simulink model "STP_1b"  (R2023a)
settings: Solver=ode4  StartTime=0.0  StopTime=30  FixedStep=0.005  RelTol=1e-3
InitFcn:
  | STP
values from neighbouring files (symbols this model uses):
  K_scheduled = zeros(length(V_op), 2)    [CAL3.m]    (also in CUB.m; DLC2.m; MUS.m; OHZ.m)
  V_op = 5:5:85    [CAL3.m]    (also in CUB.m; DLC2.m; MUS.m; OHZ.m)
  X_track = [linspace(0, runway_length, 200)'; runway_length + R_track * cos(theta_circ(2:end))]    [CAL3.m]    (also in CUB.m = [0; 5000]; DLC2.m = 0:0.1:total_track_length; MUS.m = [0; 2000]; OHZ.m = [0; 2000])
  Y_track = [zeros(200, 1); R_track + R_track * sin(theta_circ(2:end))]    [CAL3.m]    (also in CUB.m = [0; 0]; DLC2.m = zeros(size(X_track)); MUS.m = [0; 0]; OHZ.m = [0; 0])
libraries: simulink x2, slpidlib x2
(part 1 of 3)
settings Model: NumberOfSteps=1000  SnapshotBufferSize=1000  SnapshotInterval=1000  Creator=KBISWAS  LastModifiedBy=KBISWAS

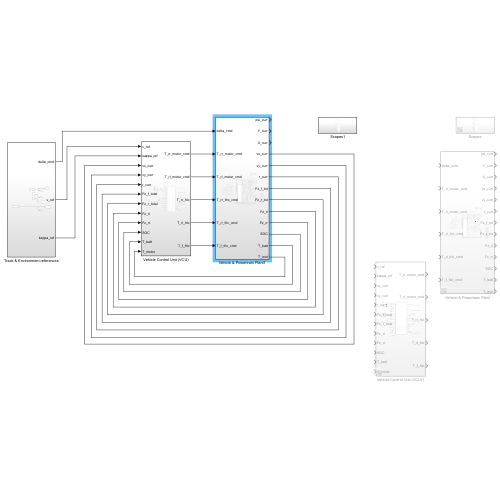
[thumbnail: Simulink's stored preview of the top-level diagram]
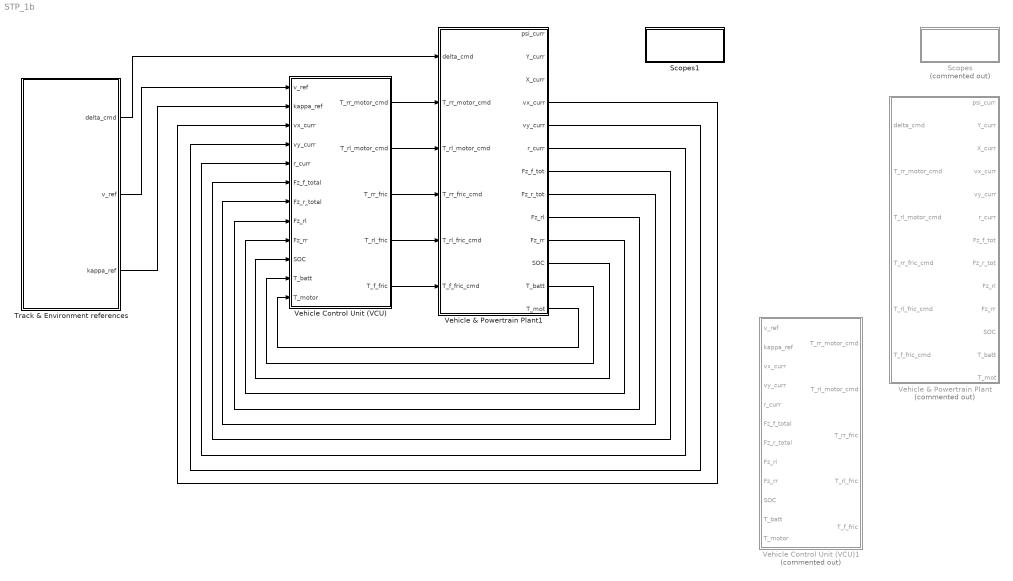
== system STP_1b ==
  Scopes : Subsystem  Commented=on
  Scopes1 : Subsystem
  Track & Environment references : Subsystem
  Vehicle & Powertrain Plant : Subsystem  Commented=on
  Vehicle & Powertrain Plant1 : Subsystem
  Vehicle Control Unit (VCU) : Subsystem
  Vehicle Control Unit (VCU)1 : Subsystem  Commented=on
  wires:
  Track & Environment references/2(v_ref) -> Vehicle Control Unit (VCU)/1(v_ref)
  Vehicle Control Unit (VCU)/1(T_rr_motor_cmd) -> Vehicle & Powertrain Plant1/2(T_rr_motor_cmd)
  Track & Environment references/3(kappa_ref) -> Vehicle Control Unit (VCU)/2(kappa_ref)
  Track & Environment references/1(delta_cmd) -> Vehicle & Powertrain Plant1/1(delta_cmd)
  Vehicle Control Unit (VCU)/2(T_rl_motor_cmd) -> Vehicle & Powertrain Plant1/3(T_rl_motor_cmd)
  Vehicle Control Unit (VCU)/3(T_rr_fric) -> Vehicle & Powertrain Plant1/4(T_rr_fric_cmd)
  Vehicle Control Unit (VCU)/4(T_rl_fric) -> Vehicle & Powertrain Plant1/5(T_rl_fric_cmd)
  Vehicle Control Unit (VCU)/5(T_f_fric) -> Vehicle & Powertrain Plant1/6(T_f_fric_cmd)
  Vehicle & Powertrain Plant1/4(vx_curr) -> Vehicle Control Unit (VCU)/3(vx_curr)
  Vehicle & Powertrain Plant1/5(vy_curr) -> Vehicle Control Unit (VCU)/4(vy_curr)
  Vehicle & Powertrain Plant1/6(r_curr) -> Vehicle Control Unit (VCU)/5(r_curr)
  Vehicle & Powertrain Plant1/7(Fz_f_tot) -> Vehicle Control Unit (VCU)/6(Fz_f_total)
  Vehicle & Powertrain Plant1/8(Fz_r_tot) -> Vehicle Control Unit (VCU)/7(Fz_r_total)
  Vehicle & Powertrain Plant1/9(Fz_rl) -> Vehicle Control Unit (VCU)/8(Fz_rl)
  Vehicle & Powertrain Plant1/10(Fz_rr) -> Vehicle Control Unit (VCU)/9(Fz_rr)
  Vehicle & Powertrain Plant1/11(SOC) -> Vehicle Control Unit (VCU)/10(SOC)
  Vehicle & Powertrain Plant1/12(T_batt) -> Vehicle Control Unit (VCU)/11(T_batt)
  Vehicle & Powertrain Plant1/13(T_mot) -> Vehicle Control Unit (VCU)/12(T_motor)

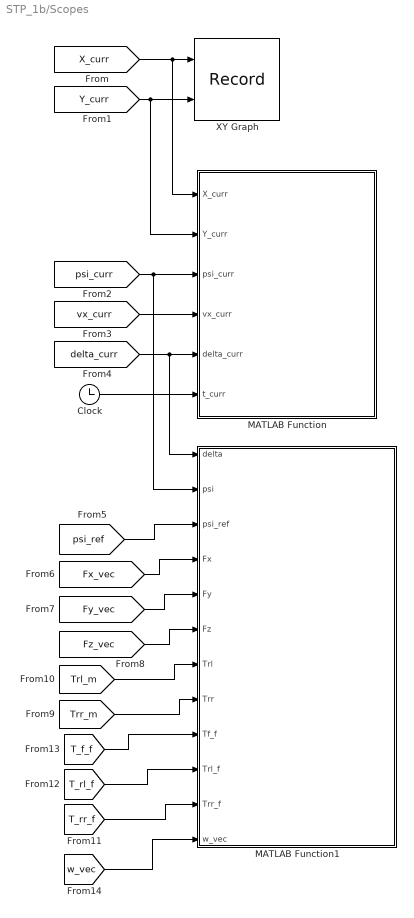
== system STP_1b/Scopes ==
  Clock : Clock
  MATLAB Function : MATLAB Function  TreatAsAtomicUnit=on
  MATLAB Function1 : MATLAB Function  TreatAsAtomicUnit=on
  XY Graph : Record  FileSettingsInternal="{\"entries\":[{\"content\":{\"excelSettings\":{\"content\":{},\"type\":\"Streamout.ExcelSettings\"}},\"type\":\"Streamout.FileSettingStorage\",\"uuid\":\"\"}],\"packageUris\":[\"http:\\/\\/schema.mathworks.com\\/mf0\\/streamout_blocks\\/R2020a\"],\"version\":\"1.0\"}"  Layout=[1 1]  SignalsInternal="{\"entries\":[{\"content\":{},\"type\":\"RecordBlkView.InputSignals\",\"uuid\":\"\"}],\"packageUris\":[\"http:\\/\\/schema.mathworks.com\\/mf0\\/streamout_blocks\\/R2020a\"],\"version\":\"1.0\"}"  VisualizationBindings="{\"xyplotplugin\":{\"info\":[{\"series\":[],\"subplotID\":1}]}}"  CompatibilityTag=XY
  wires:
  [X_curr] -> MATLAB Function/1(X_curr), XY Graph/1
  [Y_curr] -> MATLAB Function/2(Y_curr), XY Graph/2
  [psi_curr] -> MATLAB Function/3(psi_curr), MATLAB Function1/2(psi)
  [vx_curr] -> MATLAB Function/4(vx_curr)
  [delta_curr] -> MATLAB Function1/1(delta), MATLAB Function/5(delta_curr)
  Clock/1 -> MATLAB Function/6(t_curr)
  [psi_ref] -> MATLAB Function1/3(psi_ref)
  [Fx_vec] -> MATLAB Function1/4(Fx)
  [Fy_vec] -> MATLAB Function1/5(Fy)
  [Fz_vec] -> MATLAB Function1/6(Fz)
  [Trr_m] -> MATLAB Function1/8(Trr)
  [Trl_m] -> MATLAB Function1/7(Trl)
  [T_f_f] -> MATLAB Function1/9(Tf_f)
  [T_rr_f] -> MATLAB Function1/11(Trr_f)
  [T_rl_f] -> MATLAB Function1/10(Trl_f)
  [w_vec] -> MATLAB Function1/12(w_vec)

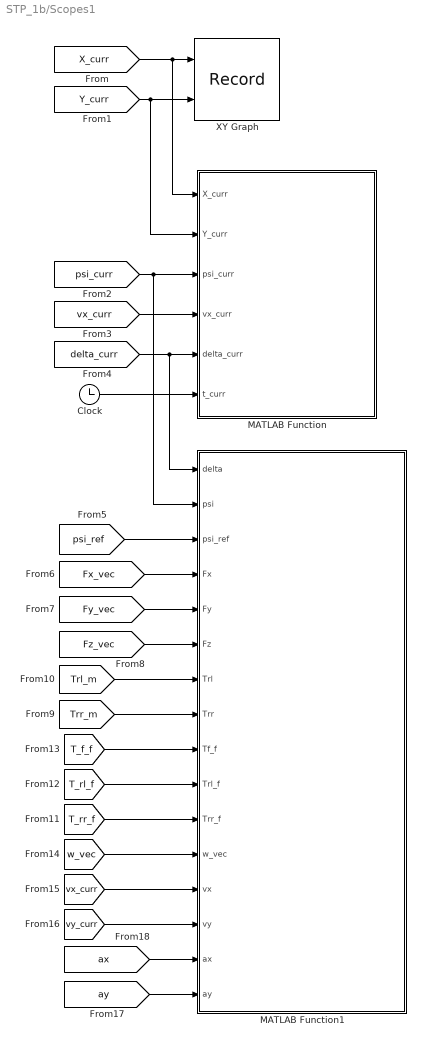
== system STP_1b/Scopes1 ==
  Clock : Clock
  MATLAB Function : MATLAB Function  TreatAsAtomicUnit=on
  MATLAB Function1 : MATLAB Function  TreatAsAtomicUnit=on
  XY Graph : Record  FileSettingsInternal="{\"entries\":[{\"content\":{\"excelSettings\":{\"content\":{},\"type\":\"Streamout.ExcelSettings\"}},\"type\":\"Streamout.FileSettingStorage\",\"uuid\":\"\"}],\"packageUris\":[\"http:\\/\\/schema.mathworks.com\\/mf0\\/streamout_blocks\\/R2020a\"],\"version\":\"1.0\"}"  Layout=[1 1]  SignalsInternal="{\"entries\":[{\"content\":{\"signals\":[{\"content\":{\"blockPath\":[],\"dimensions\":[1],\"domain\":\"\",\"lineColor\":\"#fe330a\",\"port\":1,\"sid\":[\"\"],\"signalID\":421428,\"signalName\":\"From\"},\"type\":\"RecordBlkView.Signal\",\"uuid\":\"\"},{\"content\":{\"blockPath\":[],\"dimensions\":[1],\"domain\":\"\",\"lineColor\":\"#22b573\",\"port\":2,\"sid\":[\"\"],\"signalID\":421432,\"signalName\":\"From1\"},\"type\":\"RecordBlkView.Signal\",\"uuid\":\"\"}]},\"type\":\"RecordBlkView.InputSignals\",\"uuid\":\"\"}],\"packageUris\":[\"http:\\/\\/schema.mathworks.com\\/mf0\\/streamout_blocks\\/R2020a\"],\"version\":\"1.0\"}"  VisualizationBindings="{\"xyplotplugin\":{\"info\":[{\"series\":[],\"subplotID\":1}]}}"  CompatibilityTag=XY
  wires:
  [X_curr] -> MATLAB Function/1(X_curr), XY Graph/1
  [Y_curr] -> MATLAB Function/2(Y_curr), XY Graph/2
  [psi_curr] -> MATLAB Function1/2(psi), MATLAB Function/3(psi_curr)
  [vx_curr] -> MATLAB Function/4(vx_curr)
  [delta_curr] -> MATLAB Function1/1(delta), MATLAB Function/5(delta_curr)
  Clock/1 -> MATLAB Function/6(t_curr)
  [psi_ref] -> MATLAB Function1/3(psi_ref)
  [Fx_vec] -> MATLAB Function1/4(Fx)
  [Fy_vec] -> MATLAB Function1/5(Fy)
  [Fz_vec] -> MATLAB Function1/6(Fz)
  [Trr_m] -> MATLAB Function1/8(Trr)
  [Trl_m] -> MATLAB Function1/7(Trl)
  [T_f_f] -> MATLAB Function1/9(Tf_f)
  [T_rr_f] -> MATLAB Function1/11(Trr_f)
  [T_rl_f] -> MATLAB Function1/10(Trl_f)
  [w_vec] -> MATLAB Function1/12(w_vec)
  [vx_curr] -> MATLAB Function1/13(vx)
  [vy_curr] -> MATLAB Function1/14(vy)
  [ax] -> MATLAB Function1/15(ax)
  [ay] -> MATLAB Function1/16(ay)

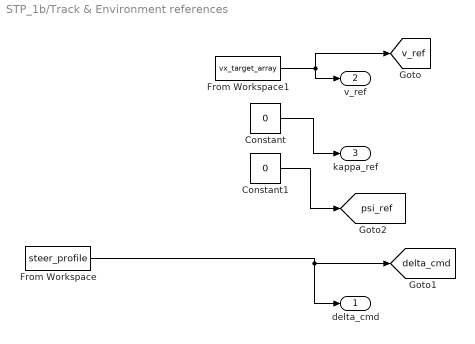
== system STP_1b/Track & Environment references ==
  Constant : Constant  Value=0
  Constant1 : Constant  Value=0
  From Workspace : FromWorkspace  VariableName=steer_profile
  From Workspace1 : FromWorkspace  VariableName=vx_target_array
  delta_cmd : Outport
  v_ref : Outport  Port=2
  kappa_ref : Outport  Port=3
  tag scope: delta_cmd=global, psi_ref=global, v_ref=global
  wires:
  From Workspace/1 -> delta_cmd/1, [delta_cmd]
  From Workspace1/1 -> v_ref/1, [v_ref]
  Constant1/1 -> [psi_ref]
  Constant/1 -> kappa_ref/1

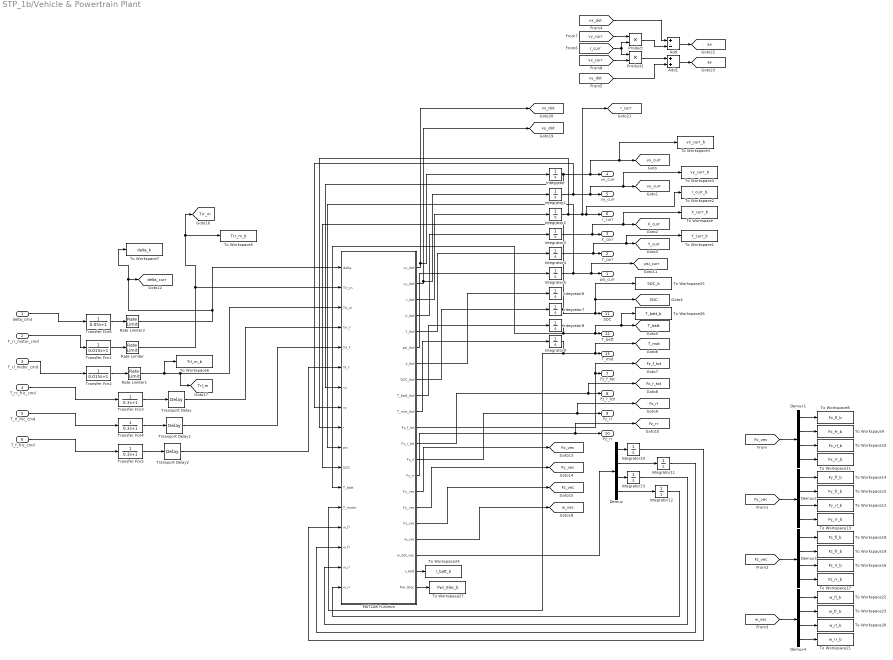
== system STP_1b/Vehicle & Powertrain Plant ==
  delta_cmd : Inport
  T_rr_motor_cmd : Inport  Port=2
  T_rl_motor_cmd : Inport  Port=3
  T_rr_fric_cmd : Inport  Port=4
  T_rl_fric_cmd : Inport  Port=5
  T_f_fric_cmd : Inport  Port=6
  Add : Sum  Inputs=+-
  Add1 : Sum
  Demux{,1..4} (5 alike) : Demux
  Integrator : Integrator  InitialCondition=5
  Integrator{1..6,10..13} (10 alike) : Integrator
  Integrator7 : Integrator  InitialCondition=0.9
  Integrator8 : Integrator  InitialCondition=30
  Integrator9 : Integrator  InitialCondition=30
  MATLAB Function : MATLAB Function  TreatAsAtomicUnit=on
  Product : Product
  Product1 : Product
  Rate Limiter : RateLimiter  RisingSlewLimit=500  FallingSlewLimit=-500  SampleTimeMode=inherited
  Rate Limiter1 : RateLimiter  RisingSlewLimit=500  FallingSlewLimit=-500  SampleTimeMode=inherited
  Rate Limiter2 : RateLimiter  RisingSlewLimit=0.05  FallingSlewLimit=-0.05  SampleTimeMode=inherited
  To Workspace : ToWorkspace  VariableName=X_curr_b  SaveFormat=Timeseries  SampleTime=-1
  To Workspace1 : ToWorkspace  VariableName=Y_curr_b  SaveFormat=Timeseries  SampleTime=-1
  To Workspace10 : ToWorkspace  VariableName=Fx_rl_b  SaveFormat=Timeseries  SampleTime=-1
  To Workspace11 : ToWorkspace  VariableName=Fx_rr_b  SaveFormat=Timeseries  SampleTime=-1
  To Workspace12 : ToWorkspace  VariableName=Fy_rl_b  SaveFormat=Timeseries  SampleTime=-1
  To Workspace13 : ToWorkspace  VariableName=Fy_rr_b  SaveFormat=Timeseries  SampleTime=-1
  To Workspace14 : ToWorkspace  VariableName=Fy_fl_b  SaveFormat=Timeseries  SampleTime=-1
  To Workspace15 : ToWorkspace  VariableName=Fy_fr_b  SaveFormat=Timeseries  SampleTime=-1
  To Workspace16 : ToWorkspace  VariableName=Fz_rl_b  SaveFormat=Timeseries  SampleTime=-1
  To Workspace17 : ToWorkspace  VariableName=Fz_rr_b  SaveFormat=Timeseries  SampleTime=-1
  To Workspace18 : ToWorkspace  VariableName=Fz_fl_b  SaveFormat=Timeseries  SampleTime=-1
  To Workspace19 : ToWorkspace  VariableName=Fz_fr_b  SaveFormat=Timeseries  SampleTime=-1
  To Workspace2 : ToWorkspace  VariableName=r_curr_b  SaveFormat=Timeseries  SampleTime=-1
  To Workspace20 : ToWorkspace  VariableName=w_rl_b  SaveFormat=Timeseries  SampleTime=-1
  To Workspace21 : ToWorkspace  VariableName=w_rr_b  SaveFormat=Timeseries  SampleTime=-1
  To Workspace22 : ToWorkspace  VariableName=w_fl_b  SaveFormat=Timeseries  SampleTime=-1
  To Workspace23 : ToWorkspace  VariableName=w_fr_b  SaveFormat=Timeseries  SampleTime=-1
  To Workspace24 : ToWorkspace  VariableName=I_batt_b  SaveFormat=Timeseries  SampleTime=-1
  To Workspace25 : ToWorkspace  VariableName=SOC_b  SaveFormat=Timeseries  SampleTime=-1
  To Workspace26 : ToWorkspace  VariableName=T_batt_b  SaveFormat=Timeseries  SampleTime=-1
  To Workspace27 : ToWorkspace  VariableName=Pwr_Elec_b  SaveFormat=Timeseries  SampleTime=-1
  To Workspace3 : ToWorkspace  VariableName=vx_curr_b  SaveFormat=Timeseries  SampleTime=-1
  To Workspace4 : ToWorkspace  VariableName=vy_curr_b  SaveFormat=Timeseries  SampleTime=-1
  To Workspace5 : ToWorkspace  VariableName=Trr_m_b  SaveFormat=Timeseries  SampleTime=-1
  To Workspace6 : ToWorkspace  VariableName=Trl_m_b  SaveFormat=Timeseries  SampleTime=-1
  To Workspace7 : ToWorkspace  VariableName=delta_b  SaveFormat=Timeseries  SampleTime=-1
  To Workspace8 : ToWorkspace  VariableName=Fx_fl_b  SaveFormat=Timeseries  SampleTime=-1
  To Workspace9 : ToWorkspace  VariableName=Fx_fr_b  SaveFormat=Timeseries  SampleTime=-1
  Transfer Fcn1 : TransferFcn  Denominator=[0.015 1]
  Transfer Fcn2 : TransferFcn  Denominator=[0.015 1]
  Transfer Fcn3 : TransferFcn  Denominator=[0.3 1]
  Transfer Fcn4 : TransferFcn  Denominator=[0.3 1]
  Transfer Fcn5 : TransferFcn  Denominator=[0.3 1]
  Transfer Fcn6 : TransferFcn  Numerator=1  Denominator=[0.05 1]
  Transport Delay : TransportDelay  DelayTime=0.03
  Transport Delay1 : TransportDelay  DelayTime=0.03
  Transport Delay2 : TransportDelay  DelayTime=0.03
  psi_curr : Outport
  Y_curr : Outport  Port=2
  X_curr : Outport  Port=3
  vx_curr : Outport  Port=4
  vy_curr : Outport  Port=5
  r_curr : Outport  Port=6
  Fz_f_tot : Outport  Port=7
  Fz_r_tot : Outport  Port=8
  Fz_rl : Outport  Port=9
  Fz_rr : Outport  Port=10
  SOC : Outport  Port=11
  T_batt : Outport  Port=12
  T_mot : Outport  Port=13
  tag scope: Fx_vec=global, Fy_vec=global, Fz_f_tot=global, Fz_r_tot=global, Fz_rl=global, Fz_rr=global, Fz_vec=global, SOC=global, T_batt=global, T_mot=global, Trl_m=global, Trr_m=global, X_curr=global, Y_curr=global, ax=global, ay=global, delta_curr=global, psi_curr=global, r_curr=global, vx_curr=global, vx_dot=global, vy_curr=global, vy_dot=global, w_vec=global
  wires:
  T_rr_fric_cmd/1 -> Transfer Fcn3/1
  T_rl_fric_cmd/1 -> Transfer Fcn4/1
  T_f_fric_cmd/1 -> Transfer Fcn5/1
  Rate Limiter2/1 -> MATLAB Function/1(delta), To Workspace7/1, [delta_curr]
  Rate Limiter/1 -> To Workspace5/1, [Trr_m], MATLAB Function/2(Trr_m)
  Rate Limiter1/1 -> To Workspace6/1, MATLAB Function/3(Trl_m), [Trl_m]
  Transfer Fcn3/1 -> Transport Delay/1
  Transfer Fcn4/1 -> Transport Delay1/1
  Transfer Fcn5/1 -> Transport Delay2/1
  MATLAB Function/3(r_dot) -> Integrator2/1
  MATLAB Function/4(X_dot) -> Integrator3/1
  MATLAB Function/5(Y_dot) -> Integrator4/1
  MATLAB Function/6(psi_dot) -> Integrator5/1
  MATLAB Function/7(s_dot) -> Integrator6/1
  MATLAB Function/8(SOC_dot) -> Integrator7/1
  Integrator/1 -> MATLAB Function/7(vx), To Workspace3/1, [vx_curr], vx_curr/1
  Integrator1/1 -> MATLAB Function/8(vy), To Workspace4/1, [vy_curr], vy_curr/1
  Integrator5/1 -> MATLAB Function/10(psi), [psi_curr], psi_curr/1
  Integrator8/1 -> MATLAB Function/12(T_batt), To Workspace26/1, [T_batt], T_batt/1
  Integrator9/1 -> MATLAB Function/13(T_motor), [T_mot], T_mot/1
  Integrator4/1 -> To Workspace1/1, [Y_curr], Y_curr/1
  Integrator3/1 -> To Workspace/1, [X_curr], X_curr/1
  MATLAB Function/11(Fz_f_tot) -> [Fz_f_tot], Fz_f_tot/1
  Integrator7/1 -> MATLAB Function/11(SOC), To Workspace25/1, [SOC], SOC/1
  MATLAB Function/14(Fz_rr) -> [Fz_rr], Fz_rr/1
  MATLAB Function/15(Fx_vec) -> [Fx_vec]
  MATLAB Function/17(Fz_vec) -> [Fz_vec]
  MATLAB Function/9(T_batt_dot) -> Integrator8/1
  MATLAB Function/10(T_mot_dot) -> Integrator9/1
  MATLAB Function/12(Fz_r_tot) -> [Fz_r_tot], Fz_r_tot/1
  MATLAB Function/13(Fz_rl) -> [Fz_rl], Fz_rl/1
  MATLAB Function/16(Fy_vec) -> [Fy_vec]
  MATLAB Function/18(w_vec) -> [w_vec]
  Demux/4 -> Integrator12/1
  Demux/3 -> Integrator13/1
  Demux/2 -> Integrator11/1
  Demux/1 -> Integrator10/1
  MATLAB Function/19(w_dot_vec) -> Demux/1
  Integrator10/1 -> MATLAB Function/14(w_fl)
  Integrator11/1 -> MATLAB Function/15(w_fr)
  Integrator12/1 -> MATLAB Function/17(w_rr)
  Integrator13/1 -> MATLAB Function/16(w_rl)
  Demux1/2 -> To Workspace9/1
  [w_vec] -> Demux4/1
  Demux3/2 -> To Workspace19/1
  Demux3/4 -> To Workspace17/1
  Demux3/3 -> To Workspace16/1
  [Fy_vec] -> Demux2/1
  Demux2/1 -> To Workspace14/1
  Demux2/3 -> To Workspace12/1
  [Fz_vec] -> Demux3/1
  Demux2/4 -> To Workspace13/1
  Demux2/2 -> To Workspace15/1
  Demux1/4 -> To Workspace11/1
  Demux1/1 -> To Workspace8/1
  Demux1/3 -> To Workspace10/1
  [Fx_vec] -> Demux1/1
  Demux3/1 -> To Workspace18/1
  Demux4/1 -> To Workspace22/1
  Demux4/4 -> To Workspace21/1
  Demux4/3 -> To Workspace20/1
  Demux4/2 -> To Workspace23/1
  Transfer Fcn1/1 -> Rate Limiter/1
  Transfer Fcn2/1 -> Rate Limiter1/1
  Product1/1 -> Add1/1
  [vy_curr] -> Product/1
  Product/1 -> Add/2
  [vx_curr] -> Product1/2
  Integrator2/1 -> [r_curr], To Workspace2/1, r_curr/1, MATLAB Function/9(r)
  MATLAB Function/1(vx_dot) -> [vx_dot], Integrator/1
  [r_curr] -> Product1/1, Product/2
  [vy_dot] -> Add1/2
  Add/1 -> [ax]
  Add1/1 -> [ay]
  [vx_dot] -> Add/1
  MATLAB Function/2(vy_dot) -> [vy_dot], Integrator1/1
  T_rr_motor_cmd/1 -> Transfer Fcn1/1
  T_rl_motor_cmd/1 -> Transfer Fcn2/1
  MATLAB Function/20(I_batt) -> To Workspace24/1
  MATLAB Function/21(Pwr_Elec) -> To Workspace27/1
  Transfer Fcn6/1 -> Rate Limiter2/1
  delta_cmd/1 -> Transfer Fcn6/1
  Transport Delay1/1 -> MATLAB Function/5(Trl_f)
  Transport Delay2/1 -> MATLAB Function/6(Tf_f)
  Transport Delay/1 -> MATLAB Function/4(Trr_f)

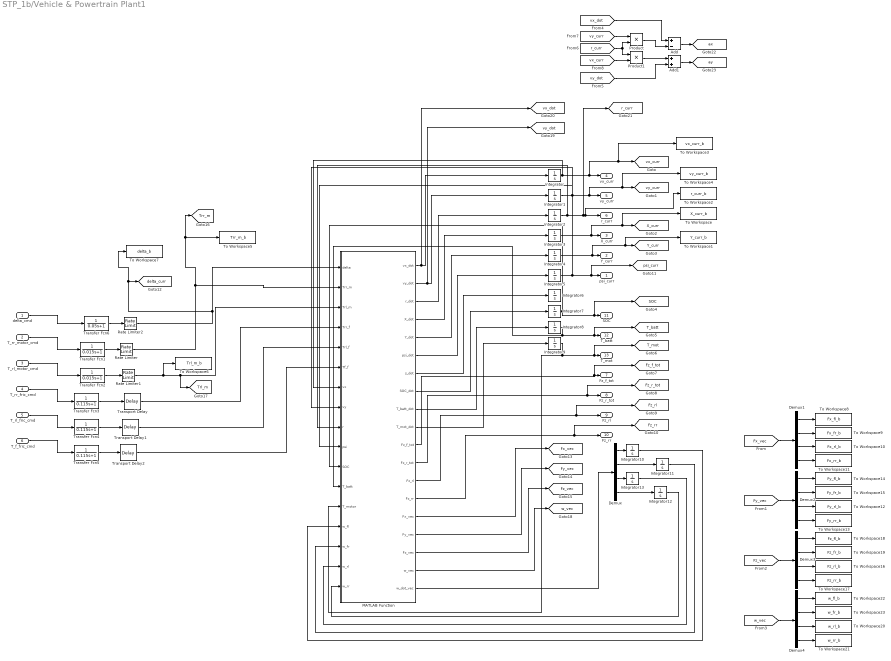
== system STP_1b/Vehicle & Powertrain Plant1 ==
  delta_cmd : Inport
  T_rr_motor_cmd : Inport  Port=2
  T_rl_motor_cmd : Inport  Port=3
  T_rr_fric_cmd : Inport  Port=4
  T_rl_fric_cmd : Inport  Port=5
  T_f_fric_cmd : Inport  Port=6
  Add : Sum  Inputs=+-
  Add1 : Sum
  Demux{,1..4} (5 alike) : Demux
  Integrator : Integrator  InitialCondition=5
  Integrator{1..6,10..13} (10 alike) : Integrator
  Integrator7 : Integrator  InitialCondition=0.9
  Integrator8 : Integrator  InitialCondition=30
  Integrator9 : Integrator  InitialCondition=30
  MATLAB Function : MATLAB Function  TreatAsAtomicUnit=on
  Product : Product
  Product1 : Product
  Rate Limiter : RateLimiter  RisingSlewLimit=500  FallingSlewLimit=-500  SampleTimeMode=inherited
  Rate Limiter1 : RateLimiter  RisingSlewLimit=500  FallingSlewLimit=-500  SampleTimeMode=inherited
  Rate Limiter2 : RateLimiter  RisingSlewLimit=0.05  FallingSlewLimit=-0.05  SampleTimeMode=inherited
  To Workspace : ToWorkspace  VariableName=X_curr_b  SaveFormat=Timeseries  SampleTime=-1
  To Workspace1 : ToWorkspace  VariableName=Y_curr_b  SaveFormat=Timeseries  SampleTime=-1
  To Workspace10 : ToWorkspace  VariableName=Fx_rl_b  SaveFormat=Timeseries  SampleTime=-1
  To Workspace11 : ToWorkspace  VariableName=Fx_rr_b  SaveFormat=Timeseries  SampleTime=-1
  To Workspace12 : ToWorkspace  VariableName=Fy_rl_b  SaveFormat=Timeseries  SampleTime=-1
  To Workspace13 : ToWorkspace  VariableName=Fy_rr_b  SaveFormat=Timeseries  SampleTime=-1
  To Workspace14 : ToWorkspace  VariableName=Fy_fl_b  SaveFormat=Timeseries  SampleTime=-1
  To Workspace15 : ToWorkspace  VariableName=Fy_fr_b  SaveFormat=Timeseries  SampleTime=-1
  To Workspace16 : ToWorkspace  VariableName=Fz_rl_b  SaveFormat=Timeseries  SampleTime=-1
  To Workspace17 : ToWorkspace  VariableName=Fz_rr_b  SaveFormat=Timeseries  SampleTime=-1
  To Workspace18 : ToWorkspace  VariableName=Fz_fl_b  SaveFormat=Timeseries  SampleTime=-1
  To Workspace19 : ToWorkspace  VariableName=Fz_fr_b  SaveFormat=Timeseries  SampleTime=-1
  To Workspace2 : ToWorkspace  VariableName=r_curr_b  SaveFormat=Timeseries  SampleTime=-1
  To Workspace20 : ToWorkspace  VariableName=w_rl_b  SaveFormat=Timeseries  SampleTime=-1
  To Workspace21 : ToWorkspace  VariableName=w_rr_b  SaveFormat=Timeseries  SampleTime=-1
  To Workspace22 : ToWorkspace  VariableName=w_fl_b  SaveFormat=Timeseries  SampleTime=-1
  To Workspace23 : ToWorkspace  VariableName=w_fr_b  SaveFormat=Timeseries  SampleTime=-1
  To Workspace3 : ToWorkspace  VariableName=vx_curr_b  SaveFormat=Timeseries  SampleTime=-1
  To Workspace4 : ToWorkspace  VariableName=vy_curr_b  SaveFormat=Timeseries  SampleTime=-1
  To Workspace5 : ToWorkspace  VariableName=Trr_m_b  SaveFormat=Timeseries  SampleTime=-1
  To Workspace6 : ToWorkspace  VariableName=Trl_m_b  SaveFormat=Timeseries  SampleTime=-1
  To Workspace7 : ToWorkspace  VariableName=delta_b  SaveFormat=Timeseries  SampleTime=-1
  To Workspace8 : ToWorkspace  VariableName=Fx_fl_b  SaveFormat=Timeseries  SampleTime=-1
  To Workspace9 : ToWorkspace  VariableName=Fx_fr_b  SaveFormat=Timeseries  SampleTime=-1
  Transfer Fcn1 : TransferFcn  Denominator=[0.015 1]
  Transfer Fcn2 : TransferFcn  Denominator=[0.015 1]
  Transfer Fcn3 : TransferFcn  Denominator=[0.115 1]
  Transfer Fcn4 : TransferFcn  Denominator=[0.115 1]
  Transfer Fcn5 : TransferFcn  Denominator=[0.115 1]
  Transfer Fcn6 : TransferFcn  Numerator=1  Denominator=[0.05 1]
  Transport Delay : TransportDelay  DelayTime=0.05
  Transport Delay1 : TransportDelay  DelayTime=0.05
  Transport Delay2 : TransportDelay  DelayTime=0.05
  psi_curr : Outport
  Y_curr : Outport  Port=2
  X_curr : Outport  Port=3
  vx_curr : Outport  Port=4
  vy_curr : Outport  Port=5
  r_curr : Outport  Port=6
  Fz_f_tot : Outport  Port=7
  Fz_r_tot : Outport  Port=8
  Fz_rl : Outport  Port=9
  Fz_rr : Outport  Port=10
  SOC : Outport  Port=11
  T_batt : Outport  Port=12
  T_mot : Outport  Port=13
  tag scope: Fx_vec=global, Fy_vec=global, Fz_f_tot=global, Fz_r_tot=global, Fz_rl=global, Fz_rr=global, Fz_vec=global, SOC=global, T_batt=global, T_mot=global, Trl_m=global, Trr_m=global, X_curr=global, Y_curr=global, ax=global, ay=global, delta_curr=global, psi_curr=global, r_curr=global, vx_curr=global, vx_dot=global, vy_curr=global, vy_dot=global, w_vec=global
  wires:
  Demux4/2 -> To Workspace23/1
  Demux4/3 -> To Workspace20/1
  Demux4/4 -> To Workspace21/1
  Demux4/1 -> To Workspace22/1
  Demux3/1 -> To Workspace18/1
  [Fx_vec] -> Demux1/1
  Demux1/3 -> To Workspace10/1
  Demux1/1 -> To Workspace8/1
  Demux1/4 -> To Workspace11/1
  Demux2/2 -> To Workspace15/1
  Demux2/4 -> To Workspace13/1
  [Fz_vec] -> Demux3/1
  Demux2/3 -> To Workspace12/1
  Demux2/1 -> To Workspace14/1
  [Fy_vec] -> Demux2/1
  Demux3/3 -> To Workspace16/1
  Demux3/4 -> To Workspace17/1
  Demux3/2 -> To Workspace19/1
  [w_vec] -> Demux4/1
  Demux1/2 -> To Workspace9/1
  Integrator13/1 -> MATLAB Function/16(w_rl)
  Integrator12/1 -> MATLAB Function/17(w_rr)
  Integrator11/1 -> MATLAB Function/15(w_fr)
  Integrator10/1 -> MATLAB Function/14(w_fl)
  MATLAB Function/19(w_dot_vec) -> Demux/1
  Demux/1 -> Integrator10/1
  Demux/2 -> Integrator11/1
  Demux/3 -> Integrator13/1
  Demux/4 -> Integrator12/1
  MATLAB Function/18(w_vec) -> [w_vec]
  MATLAB Function/16(Fy_vec) -> [Fy_vec]
  MATLAB Function/13(Fz_rl) -> Fz_rl/1, [Fz_rl]
  MATLAB Function/12(Fz_r_tot) -> Fz_r_tot/1, [Fz_r_tot]
  MATLAB Function/10(T_mot_dot) -> Integrator9/1
  MATLAB Function/9(T_batt_dot) -> Integrator8/1
  MATLAB Function/17(Fz_vec) -> [Fz_vec]
  MATLAB Function/15(Fx_vec) -> [Fx_vec]
  MATLAB Function/14(Fz_rr) -> Fz_rr/1, [Fz_rr]
  Integrator7/1 -> SOC/1, [SOC], MATLAB Function/11(SOC)
  MATLAB Function/11(Fz_f_tot) -> Fz_f_tot/1, [Fz_f_tot]
  Integrator3/1 -> X_curr/1, [X_curr], To Workspace/1
  Integrator4/1 -> Y_curr/1, [Y_curr], To Workspace1/1
  Integrator9/1 -> T_mot/1, [T_mot], MATLAB Function/13(T_motor)
  Integrator8/1 -> T_batt/1, [T_batt], MATLAB Function/12(T_batt)
  Integrator5/1 -> psi_curr/1, [psi_curr], MATLAB Function/10(psi)
  Integrator1/1 -> vy_curr/1, [vy_curr], To Workspace4/1, MATLAB Function/8(vy)
  Integrator/1 -> vx_curr/1, [vx_curr], To Workspace3/1, MATLAB Function/7(vx)
  MATLAB Function/8(SOC_dot) -> Integrator7/1
  MATLAB Function/7(s_dot) -> Integrator6/1
  MATLAB Function/6(psi_dot) -> Integrator5/1
  MATLAB Function/5(Y_dot) -> Integrator4/1
  MATLAB Function/4(X_dot) -> Integrator3/1
  MATLAB Function/3(r_dot) -> Integrator2/1
  Transport Delay2/1 -> MATLAB Function/6(Tf_f)
  Transport Delay1/1 -> MATLAB Function/5(Trl_f)
  Transport Delay/1 -> MATLAB Function/4(Trr_f)
  Rate Limiter1/1 -> [Trl_m], MATLAB Function/3(Trl_m), To Workspace6/1
  Rate Limiter/1 -> [Trr_m], To Workspace5/1, MATLAB Function/2(Trr_m)
  Rate Limiter2/1 -> [delta_curr], To Workspace7/1, MATLAB Function/1(delta)
  T_f_fric_cmd/1 -> Transfer Fcn5/1
  T_rl_fric_cmd/1 -> Transfer Fcn4/1
  T_rr_fric_cmd/1 -> Transfer Fcn3/1
  T_rl_motor_cmd/1 -> Transfer Fcn2/1
  T_rr_motor_cmd/1 -> Transfer Fcn1/1
  delta_cmd/1 -> Transfer Fcn6/1
  Transfer Fcn1/1 -> Rate Limiter/1
  Transfer Fcn2/1 -> Rate Limiter1/1
  Transfer Fcn6/1 -> Rate Limiter2/1
  Product1/1 -> Add1/1
  Add/1 -> [ax]
  Add1/1 -> [ay]
  [vy_dot] -> Add1/2
  MATLAB Function/2(vy_dot) -> [vy_dot], Integrator1/1
  [vx_dot] -> Add/1
  Product/1 -> Add/2
  [vx_curr] -> Product1/2
  Integrator2/1 -> MATLAB Function/9(r), [r_curr], r_curr/1, To Workspace2/1
  [r_curr] -> Product1/1, Product/2
  MATLAB Function/1(vx_dot) -> [vx_dot], Integrator/1
  [vy_curr] -> Product/1
  Transfer Fcn5/1 -> Transport Delay2/1
  Transfer Fcn4/1 -> Transport Delay1/1
  Transfer Fcn3/1 -> Transport Delay/1

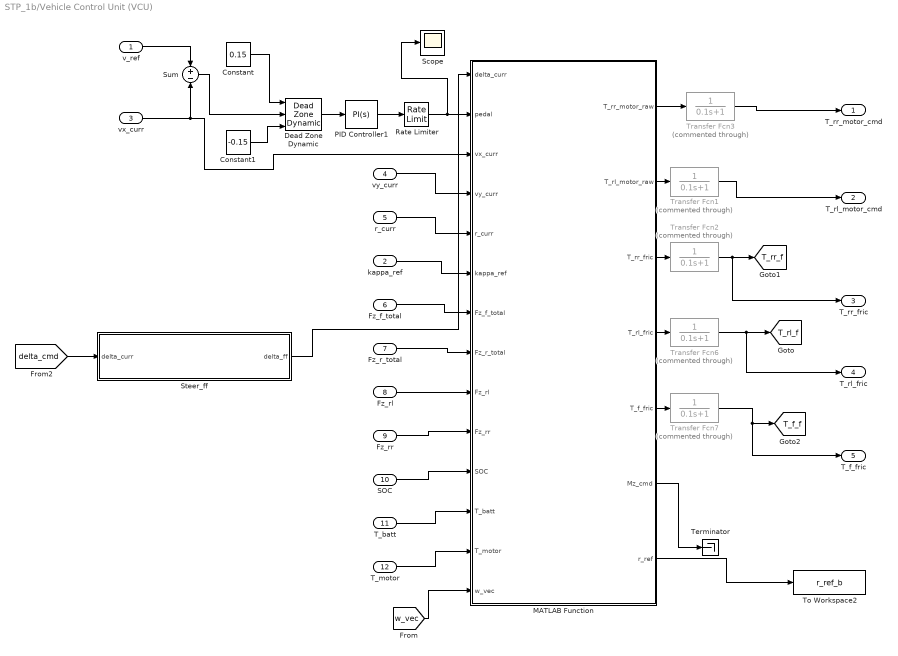
== system STP_1b/Vehicle Control Unit (VCU) ==
  v_ref : Inport
  kappa_ref : Inport  Port=2
  vx_curr : Inport  Port=3
  vy_curr : Inport  Port=4
  r_curr : Inport  Port=5
  Fz_f_total : Inport  Port=6
  Fz_r_total : Inport  Port=7
  Fz_rl : Inport  Port=8
  Fz_rr : Inport  Port=9
  SOC : Inport  Port=10
  T_batt : Inport  Port=11
  T_motor : Inport  Port=12
  Constant : Constant  Value=0.15
  Constant1 : Constant  Value=-0.15
  Dead Zone Dynamic : simulink/Discontinuities/Dead Zone Dynamic
  MATLAB Function : MATLAB Function  TreatAsAtomicUnit=on
  PID Controller1 : slpidlib/PID Controller  Controller=PI  Form=Parallel  TimeDomain=Continuous-time  UseExternalTs=off  SampleTime=-1  IntegratorMethod=Forward Euler  FilterMethod=Forward Euler  ControllerParametersSource=internal  P=0.2  I=0.5  UseKiTs=off  D=0  N=100  UseFilter=on  TunerSelectOption=Transfer Function Based (PID Tuner App)  InitialConditionSource=internal  InitialConditionForIntegrator=0  InitialConditionForFilter=0  DifferentiatorICPrevScaledInput=0  ExternalReset=none  TrackingMode=off  Kt=1  LimitOutput=on  SatLimitsSource=internal  UpperSaturationLimit=1  LowerSaturationLimit=-1  LinearizeAsGain=on  AntiWindupMode=clamping  Kb=1  LimitIntegrator=off  UpperIntegratorSaturationLimit=inf  LowerIntegratorSaturationLimit=-inf  POutMin=[]  POutMax=[]  IOutMin=[]  IOutMax=[]  DOutMin=[]  DOutMax=[]  NOutMin=[]  NOutMax=[]  SumOutMin=[]  SumOutMax=[]  SaturationOutMin=[]  SaturationOutMax=[]  PParamMin=[]  PParamMax=[]  IParamMin=[]  IParamMax=[]  DParamMin=[]  DParamMax=[]  NParamMin=[]  NParamMax=[]  KbParamMin=[]  KbParamMax=[]  KtParamMin=[]  KtParamMax=[]  KbOutMin=[]  KbOutMax=[]  KtOutMin=[]  KtOutMax=[]  IntegratorOutMin=[]  IntegratorOutMax=[]  FilterOutMin=[]  FilterOutMax=[]  SumI1OutMin=[]  SumI1OutMax=[]  SumI2OutMin=[]  SumI2OutMax=[]  SumI3OutMin=[]  SumI3OutMax=[]  SumI4OutMin=[]  SumI4OutMax=[]  SumDOutMin=[]  SumDOutMax=[]  DifferentiatorOutMin=[]  DifferentiatorOutMax=[]  FilterDiffOutCoefMin=[]  FilterDiffOutCoefMax=[]  ReciprocalOutMin=[]  ReciprocalOutMax=[]  SumDenOutMin=[]  SumDenOutMax=[]  SumNumOutMin=[]  SumNumOutMax=[]  DivideOutMin=[]  DivideOutMax=[]  UdiffTsProdOutMin=[]  UdiffTsProdOutMax=[]  NTsProdOutMin=[]  NTsProdOutMax=[]  UintegralTsProdOutMin=[]  UintegralTsProdOutMax=[]  UngainTsProdOutMin=[]  UngainTsProdOutMax=[]  ClampingZeroOutDataTypeStr=Inherit: Inherit via back propagation  ClampingZeroOutMin=[]  ClampingZeroOutMax=[]  FilterDenConstantOutDataTypeStr=Inherit: Inherit via back propagation  FilterDenConstantOutMin=[]  FilterDenConstantOutMax=[]  PCopyOutDataTypeStr=Inherit: Inherit via back propagation  PCopyOutMin=[]  PCopyOutMax=[]  NCopyOutDataTypeStr=Inherit: Inherit via back propagation  NCopyOutMin=[]  NCopyOutMax=[]  IntegratorContinuousStateAttributes=''  IntegratorStateMustResolveToSignalObject=off  IntegratorRTWStateStorageClass=Auto  FilterContinuousStateAttributes=''  FilterStateMustResolveToSignalObject=off  FilterRTWStateStorageClass=Auto  ParallelPVariant=InternalParameters  IdealPVariant=Disabled  IVariant=InternalParameters  DVariant=Disabled  IntegratorVariant=Continuous  SatVariant=Enabled  AWVariant=ContClampingParallel  PCopyVariant=Disabled  TRVariant=Disabled  FdbkBlocksVariant=Forward  IdealPFdbkVariant=Disabled  SatFdbkVariant=Disabled  DerivativeFilterVariant=Disabled  NVariant=Disabled  NCopyVariant=Disabled_SignalSpec  FilterICVariant=Disabled  IntegratorICVariant=InternalICs  ExternalResetVariant=Disabled  TRSumVariant=Passthrough  SumFdbkVariant=Disabled  SumVariant=Sum_PI  TsampFilterVariant=InternalTs  TsampNgainVariant=Passthrough  TsampIntegralVariant=Disabled_SignalSpec  ExternalSaturationOutDataTypeStr=Inherit: Same as second input
  Rate Limiter : RateLimiter  RisingSlewLimit=0.5  FallingSlewLimit=-4  SampleTimeMode=inherited
  Scope : Scope
  Steer_ff : Subsystem
  Sum : Sum  Inputs=+-
  Terminator : Terminator
  To Workspace2 : ToWorkspace  VariableName=r_ref_b  SaveFormat=Timeseries  SampleTime=-1
  Transfer Fcn{1..3,6..7} (5 alike) : TransferFcn  Commented=through  Denominator=[0.1 1]
  T_rr_motor_cmd : Outport
  T_rl_motor_cmd : Outport  Port=2
  T_rr_fric : Outport  Port=3
  T_rl_fric : Outport  Port=4
  T_f_fric : Outport  Port=5
  tag scope: T_f_f=global, T_rl_f=global, T_rr_f=global
  wires:
  v_ref/1 -> Sum/1
  vx_curr/1 -> MATLAB Function/3(vx_curr), Sum/2
  vy_curr/1 -> MATLAB Function/4(vy_curr)
  r_curr/1 -> MATLAB Function/5(r_curr)
  kappa_ref/1 -> MATLAB Function/6(kappa_ref)
  Fz_f_total/1 -> MATLAB Function/7(Fz_f_total)
  MATLAB Function/1(T_rr_motor_raw) -> Transfer Fcn3/1
  MATLAB Function/2(T_rl_motor_raw) -> Transfer Fcn1/1
  MATLAB Function/3(T_rr_fric) -> Transfer Fcn2/1
  MATLAB Function/4(T_rl_fric) -> Transfer Fcn6/1
  MATLAB Function/5(T_f_fric) -> Transfer Fcn7/1
  MATLAB Function/6(Mz_cmd) -> Terminator/1
  MATLAB Function/7(r_ref) -> To Workspace2/1
  Steer_ff/1(delta_ff) -> MATLAB Function/1(delta_curr)
  [delta_cmd] -> Steer_ff/1(delta_curr)
  Fz_r_total/1 -> MATLAB Function/8(Fz_r_total)
  Fz_rl/1 -> MATLAB Function/9(Fz_rl)
  Fz_rr/1 -> MATLAB Function/10(Fz_rr)
  SOC/1 -> MATLAB Function/11(SOC)
  T_batt/1 -> MATLAB Function/12(T_batt)
  T_motor/1 -> MATLAB Function/13(T_motor)
  [w_vec] -> MATLAB Function/14(w_vec)
  Transfer Fcn3/1 -> T_rr_motor_cmd/1
  Transfer Fcn1/1 -> T_rl_motor_cmd/1
  Transfer Fcn2/1 -> T_rr_fric/1, [T_rr_f]
  Transfer Fcn6/1 -> T_rl_fric/1, [T_rl_f]
  Transfer Fcn7/1 -> T_f_fric/1, [T_f_f]
  Dead Zone Dynamic/1 -> PID Controller1/1
  Sum/1 -> Dead Zone Dynamic/2
  Constant1/1 -> Dead Zone Dynamic/3
  PID Controller1/1 -> Rate Limiter/1
  Constant/1 -> Dead Zone Dynamic/1
  Rate Limiter/1 -> Scope/1, MATLAB Function/2(pedal)

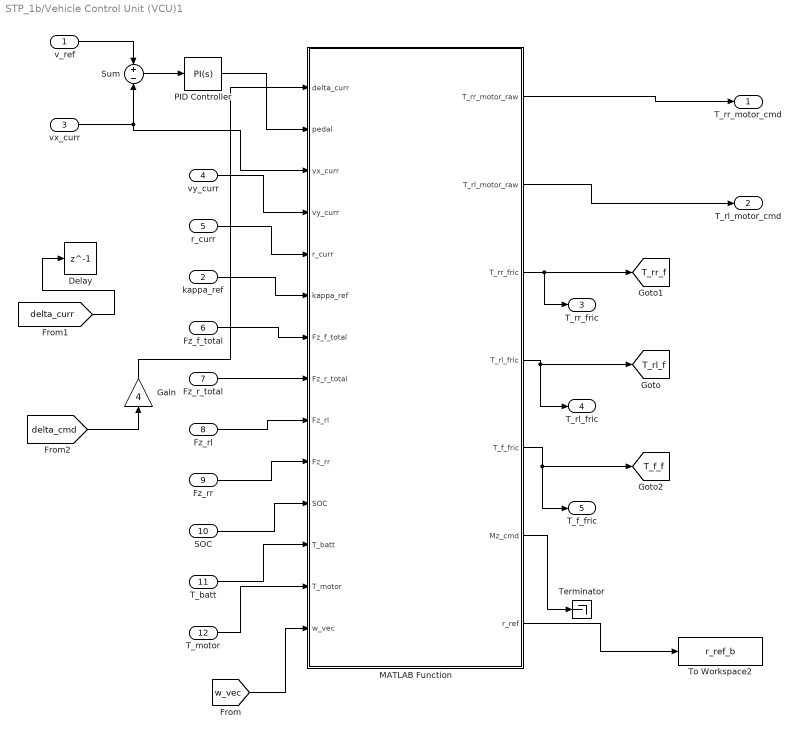
== system STP_1b/Vehicle Control Unit (VCU)1 ==
  v_ref : Inport
  kappa_ref : Inport  Port=2
  vx_curr : Inport  Port=3
  vy_curr : Inport  Port=4
  r_curr : Inport  Port=5
  Fz_f_total : Inport  Port=6
  Fz_r_total : Inport  Port=7
  Fz_rl : Inport  Port=8
  Fz_rr : Inport  Port=9
  SOC : Inport  Port=10
  T_batt : Inport  Port=11
  T_motor : Inport  Port=12
  Delay : Delay  DelayLength=1
  Gain : Gain  Gain=4
  MATLAB Function : MATLAB Function  TreatAsAtomicUnit=on
  PID Controller : slpidlib/PID Controller  Controller=PI  Form=Parallel  TimeDomain=Continuous-time  UseExternalTs=off  SampleTime=-1  IntegratorMethod=Forward Euler  FilterMethod=Forward Euler  ControllerParametersSource=internal  P=5  I=0.1  UseKiTs=off  D=0  N=100  UseFilter=on  TunerSelectOption=Transfer Function Based (PID Tuner App)  InitialConditionSource=internal  InitialConditionForIntegrator=0  InitialConditionForFilter=0  DifferentiatorICPrevScaledInput=0  ExternalReset=none  TrackingMode=off  Kt=1  LimitOutput=on  SatLimitsSource=internal  UpperSaturationLimit=1  LowerSaturationLimit=-1  LinearizeAsGain=on  AntiWindupMode=clamping  Kb=1  LimitIntegrator=off  UpperIntegratorSaturationLimit=inf  LowerIntegratorSaturationLimit=-inf  POutMin=[]  POutMax=[]  IOutMin=[]  IOutMax=[]  DOutMin=[]  DOutMax=[]  NOutMin=[]  NOutMax=[]  SumOutMin=[]  SumOutMax=[]  SaturationOutMin=[]  SaturationOutMax=[]  PParamMin=[]  PParamMax=[]  IParamMin=[]  IParamMax=[]  DParamMin=[]  DParamMax=[]  NParamMin=[]  NParamMax=[]  KbParamMin=[]  KbParamMax=[]  KtParamMin=[]  KtParamMax=[]  KbOutMin=[]  KbOutMax=[]  KtOutMin=[]  KtOutMax=[]  IntegratorOutMin=[]  IntegratorOutMax=[]  FilterOutMin=[]  FilterOutMax=[]  SumI1OutMin=[]  SumI1OutMax=[]  SumI2OutMin=[]  SumI2OutMax=[]  SumI3OutMin=[]  SumI3OutMax=[]  SumI4OutMin=[]  SumI4OutMax=[]  SumDOutMin=[]  SumDOutMax=[]  DifferentiatorOutMin=[]  DifferentiatorOutMax=[]  FilterDiffOutCoefMin=[]  FilterDiffOutCoefMax=[]  ReciprocalOutMin=[]  ReciprocalOutMax=[]  SumDenOutMin=[]  SumDenOutMax=[]  SumNumOutMin=[]  SumNumOutMax=[]  DivideOutMin=[]  DivideOutMax=[]  UdiffTsProdOutMin=[]  UdiffTsProdOutMax=[]  NTsProdOutMin=[]  NTsProdOutMax=[]  UintegralTsProdOutMin=[]  UintegralTsProdOutMax=[]  UngainTsProdOutMin=[]  UngainTsProdOutMax=[]  ClampingZeroOutDataTypeStr=Inherit: Inherit via back propagation  ClampingZeroOutMin=[]  ClampingZeroOutMax=[]  FilterDenConstantOutDataTypeStr=Inherit: Inherit via back propagation  FilterDenConstantOutMin=[]  FilterDenConstantOutMax=[]  PCopyOutDataTypeStr=Inherit: Inherit via back propagation  PCopyOutMin=[]  PCopyOutMax=[]  NCopyOutDataTypeStr=Inherit: Inherit via back propagation  NCopyOutMin=[]  NCopyOutMax=[]  IntegratorContinuousStateAttributes=''  IntegratorStateMustResolveToSignalObject=off  IntegratorRTWStateStorageClass=Auto  FilterContinuousStateAttributes=''  FilterStateMustResolveToSignalObject=off  FilterRTWStateStorageClass=Auto  ParallelPVariant=InternalParameters  IdealPVariant=Disabled  IVariant=InternalParameters  DVariant=Disabled  IntegratorVariant=Continuous  SatVariant=Enabled  AWVariant=ContClampingParallel  PCopyVariant=Disabled  TRVariant=Disabled  FdbkBlocksVariant=Forward  IdealPFdbkVariant=Disabled  SatFdbkVariant=Disabled  DerivativeFilterVariant=Disabled  NVariant=Disabled  NCopyVariant=Disabled_SignalSpec  FilterICVariant=Disabled  IntegratorICVariant=InternalICs  ExternalResetVariant=Disabled  TRSumVariant=Passthrough  SumFdbkVariant=Disabled  SumVariant=Sum_PI  TsampFilterVariant=InternalTs  TsampNgainVariant=Passthrough  TsampIntegralVariant=Disabled_SignalSpec  ExternalSaturationOutDataTypeStr=Inherit: Same as second input
  Sum : Sum  Inputs=+-
  Terminator : Terminator
  To Workspace2 : ToWorkspace  VariableName=r_ref_b  SaveFormat=Timeseries  SampleTime=-1
  T_rr_motor_cmd : Outport
  T_rl_motor_cmd : Outport  Port=2
  T_rr_fric : Outport  Port=3
  T_rl_fric : Outport  Port=4
  T_f_fric : Outport  Port=5
  tag scope: T_f_f=global, T_rl_f=global, T_rr_f=global
  wires:
  Gain/1 -> MATLAB Function/1(delta_curr)
  MATLAB Function/7(r_ref) -> To Workspace2/1
  [delta_cmd] -> Gain/1
  [delta_curr] -> Delay/1
  [w_vec] -> MATLAB Function/14(w_vec)
  MATLAB Function/6(Mz_cmd) -> Terminator/1
  MATLAB Function/5(T_f_fric) -> [T_f_f], T_f_fric/1
  MATLAB Function/4(T_rl_fric) -> [T_rl_f], T_rl_fric/1
  MATLAB Function/3(T_rr_fric) -> [T_rr_f], T_rr_fric/1
  MATLAB Function/2(T_rl_motor_raw) -> T_rl_motor_cmd/1
  MATLAB Function/1(T_rr_motor_raw) -> T_rr_motor_cmd/1
  PID Controller/1 -> MATLAB Function/2(pedal)
  T_motor/1 -> MATLAB Function/13(T_motor)
  T_batt/1 -> MATLAB Function/12(T_batt)
  SOC/1 -> MATLAB Function/11(SOC)
  Fz_rr/1 -> MATLAB Function/10(Fz_rr)
  Fz_rl/1 -> MATLAB Function/9(Fz_rl)
  Fz_r_total/1 -> MATLAB Function/8(Fz_r_total)
  Fz_f_total/1 -> MATLAB Function/7(Fz_f_total)
  kappa_ref/1 -> MATLAB Function/6(kappa_ref)
  r_curr/1 -> MATLAB Function/5(r_curr)
  vy_curr/1 -> MATLAB Function/4(vy_curr)
  Sum/1 -> PID Controller/1
  vx_curr/1 -> Sum/2, MATLAB Function/3(vx_curr)
  v_ref/1 -> Sum/1

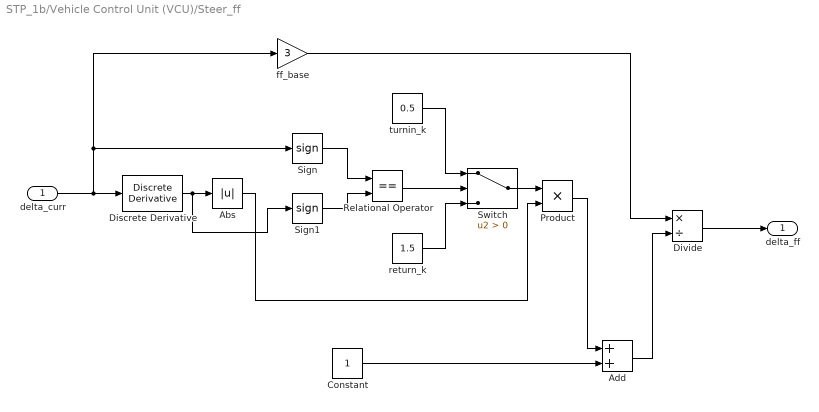
== system STP_1b/Vehicle Control Unit (VCU)/Steer_ff ==
  delta_curr : Inport
  Abs : Abs  SaturateOnIntegerOverflow=off
  Add : Sum
  Constant : Constant
  Discrete Derivative : simulink/Discrete/Discrete Derivative  gainval=1.0  ICPrevScaledInput=0.0  OutMin=[]  OutMax=[]  OutDataType=fixdt(1, 16)  OutScaling=2^-10  DoSatur=off
  Divide : Product  Inputs=*/
  Product : Product
  Relational Operator : RelationalOperator  Operator===  OutDataTypeStr=boolean  RndMeth=Simplest  InputSameDT=off
  Sign : Signum
  Sign1 : Signum
  Switch : Switch  Criteria=u2 > Threshold  SaturateOnIntegerOverflow=off  InputSameDT=off
  ff_base : Gain  Gain=3
  return_k : Constant  Value=1.5
  turnin_k : Constant  Value=0.5
  delta_ff : Outport
  wires:
  ff_base/1 -> Divide/1
  return_k/1 -> Switch/3
  Switch/1 -> Product/1
  Product/1 -> Add/1
  Sign/1 -> Relational Operator/1
  delta_curr/1 -> Discrete Derivative/1, ff_base/1, Sign/1
  Relational Operator/1 -> Switch/2
  Add/1 -> Divide/2
  Discrete Derivative/1 -> Sign1/1, Abs/1
  Abs/1 -> Product/2
  Constant/1 -> Add/2
  Sign1/1 -> Relational Operator/2
  Divide/1 -> delta_ff/1
  turnin_k/1 -> Switch/1

== matlab function STP_1b/Vehicle & Powertrain Plant/MATLAB Function ==
  data: delta input; Trr_m input; Trl_m input; Trr_f input; Trl_f input; Tf_f input; vx input; vy input; r input; psi input; SOC input; T_batt input; T_motor input; w_fl input; w_fr input; w_rl input; w_rr input; vx_dot output; vy_dot output; r_dot output; X_dot output; Y_dot output; psi_dot output; s_dot output; SOC_dot output; T_batt_dot output; T_mot_dot output; Fz_f_tot output; Fz_r_tot output; Fz_rl output; Fz_rr output; Fx_vec output; Fy_vec output; Fz_vec output; w_vec output; w_dot_vec output; veh_params parameter; I_batt output; Pwr_Elec output
function [vx_dot, vy_dot, r_dot, X_dot, Y_dot, psi_dot, s_dot, SOC_dot, T_batt_dot, T_mot_dot, Fz_f_tot, Fz_r_tot, Fz_rl, Fz_rr, Fx_vec, Fy_vec, Fz_vec, w_vec, w_dot_vec, I_batt, Pwr_Elec] = vehicle_physics_engine(delta, Trr_m, Trl_m, Trr_f, Trl_f, Tf_f, vx, vy, r, psi, SOC, T_batt, T_motor, w_fl, w_fr, w_rl, w_rr, veh_params)
    
    % =========================================================================
    % 0. EXPLICIT OUTPUT INITIALIZATION & SCALAR COERCION 
    % =========================================================================
    vx_dot = 0.0; vy_dot = 0.0; r_dot = 0.0; 
    X_dot = 0.0; Y_dot = 0.0; psi_dot = 0.0; s_dot = 0.0;
    SOC_dot = 0.0; T_batt_dot = 0.0; T_mot_dot = 0.0;
    Fz_f_tot = 0.0; Fz_r_tot = 0.0; Fz_rl = 0.0; Fz_rr = 0.0;
    Fx_vec = zeros(1,4); Fy_vec = zeros(1,4); Fz_vec = zeros(1,4);
    w_vec = zeros(1,4); w_dot_vec = zeros(1,4);
    I_batt = 0.0; 
    Pwr_Elec = 0.0; % NEW: Output initialization for Electrical Power

    % Force scalar inputs (strips undefined array dimensions from Simulink lines)
    delta = delta(1); vx = vx(1); vy = vy(1); r = r(1); psi = psi(1);
    Trr_m = Trr_m(1); Trl_m = Trl_m(1); Trr_f = Trr_f(1); Trl_f = Trl_f(1); Tf_f = Tf_f(1);
    SOC = SOC(1); T_batt = T_batt(1); T_motor = T_motor(1);
    w_fl = w_fl(1); w_fr = w_fr(1); w_rl = w_rl(1); w_rr = w_rr(1);

    % =========================================================================
    % HIGH-FIDELITY EV VEHICLE DYNAMICS PLANT MODEL
    % =========================================================================
    
    % ---------------------------------------------------------------------
    % 1. UNPACK CENTRALIZED PARAMETERS
    % ---------------------------------------------------------------------
    m = veh_params.m(1); Iz = veh_params.Iz(1); lf = veh_params.lf(1); lr = veh_params.lr(1); L = veh_params.L(1);
    tw = veh_params.tw(1); h_cg = veh_params.h_cg(1); Rw = veh_params.Rw(1); Iw = veh_params.Iw(1); 
    G = veh_params.G(1); g = veh_params.g(1); rho = veh_params.rho(1); CdA = veh_params.CdA(1);
    roll_bias_f = veh_params.roll_bias_f(1); 
    
    mu_max = veh_params.mu_max(1); C_rr = veh_params.C_rr(1);
    ks_f = veh_params.ks_f(1)/2; ks_r = veh_params.ks_r(1)/2;
    C_tire = veh_params.C_tire(1); E_tire = veh_params.E_tire(1);
    
    if abs(vx) < 0.5
        vx_safe = 0.5 * sign(vx + 1e-6); 
    else
        vx_safe = vx;
    end
    
    F_aero_drag = 0.5 * rho * CdA * vx_safe * abs(vx_safe);
    
    % ---------------------------------------------------------------------
    % 2. DYNAMIC TIRE PEAK CALIBRATION
    % ---------------------------------------------------------------------
    Fz_axle_f_static = m * g * (lr / L); 
    Fz_axle_r_static = m * g * (lf / L); 
    
    D_tire_f = mu_max * (Fz_axle_f_static / 2); 
    D_tire_r = mu_max * (Fz_axle_r_static / 2); 
    
    B_tire_f = ks_f / (C_tire * D_tire_f * 2); 
    B_tire_r = ks_r / (C_tire * D_tire_r * 2); 
    
    % ---------------------------------------------------------------------
    % 3. 3D WEIGHT TRANSFER 
    % ---------------------------------------------------------------------
    Trr_tot = Trr_m * G + Trr_f;
    Trl_tot = Trl_m * G + Trl_f;
    Tf_tot_half = Tf_f / 2; 
    
    Fx_fl_tq = Tf_tot_half / Rw; Fx_fr_tq = Tf_tot_half / Rw;
    Fx_rl_tq = Trl_tot / Rw; Fx_rr_tq = Trr_tot / Rw;
    
    ax_est = ((Fx_fl_tq + Fx_fr_tq + Fx_rl_tq + Fx_rr_tq) - F_aero_drag) / m;
    ay_est = vx_safe * r;
    
    Fz_f_tot = m * g * (lr / L) - m * ax_est * (h_cg / L);
    Fz_r_tot = m * g * (lf / L) + m * ax_est * (h_cg / L);
    
    dFz_y_f = m * ay_est * (h_cg / tw) * roll_bias_f;
    dFz_y_r = m * ay_est * (h_cg / tw) * (1 - roll_bias_f);
    
    Fz_max_f = Fz_axle_f_static * 2.5; 
    Fz_max_r = Fz_axle_r_static * 2.5;
    
    Fz_fl = max(100, min(Fz_max_f, Fz_f_tot / 2 - dFz_y_f));
    Fz_fr = max(100, min(Fz_max_f, Fz_f_tot / 2 + dFz_y_f));
    Fz_rl = max(100, min(Fz_max_r, Fz_r_tot / 2 - dFz_y_r));
    Fz_rr = max(100, min(Fz_max_r, Fz_r_tot / 2 + dFz_y_r));
    Fz_vec = [Fz_fl, Fz_fr, Fz_rl, Fz_rr];
    
    % ---------------------------------------------------------------------
    % 4. VECTOR-SUM PACEJKA COMBINED SLIP MODEL
    % ---------------------------------------------------------------------
    v_hub_fl = vx_safe - (tw / 2) * r; v_hub_fr = vx_safe + (tw / 2) * r;
    v_hub_rl = vx_safe - (tw / 2) * r; v_hub_rr = vx_safe + (tw / 2) * r;
    
    k_fl = (w_fl * Rw - v_hub_fl) / max(abs(v_hub_fl), 1.0);
    k_fr = (w_fr * Rw - v_hub_fr) / max(abs(v_hub_fr), 1.0);
    k_rl = (w_rl * Rw - v_hub_rl) / max(abs(v_hub_rl), 1.0);
    k_rr = (w_rr * Rw - v_hub_rr) / max(abs(v_hub_rr), 1.0);
    
    alpha_fl = delta - atan((vy + lf * r) / max(abs(v_hub_fl), 1.0));
    alpha_fr = delta - atan((vy + lf * r) / max(abs(v_hub_fr), 1.0));
    alpha_rl = -atan((vy - lr * r) / max(abs(v_hub_rl), 1.0));
    alpha_rr = -atan((vy - lr * r) / max(abs(v_hub_rr), 1.0));
    
    sigma_fl = sqrt(k_fl^2 + tan(alpha_fl)^2) + 1e-6;
    sigma_fr = sqrt(k_fr^2 + tan(alpha_fr)^2) + 1e-6;
    sigma_rl = sqrt(k_rl^2 + tan(alpha_rl)^2) + 1e-6;
    sigma_rr = sqrt(k_rr^2 + tan(alpha_rr)^2) + 1e-6;
    
    F_tot_fl = mu_max * Fz_fl * sin(C_tire * atan(B_tire_f * sigma_fl - E_tire * (B_tire_f * sigma_fl - atan(B_tire_f * sigma_fl))));
    F_tot_fr = mu_max * Fz_fr * sin(C_tire * atan(B_tire_f * sigma_fr - E_tire * (B_tire_f * sigma_fr - atan(B_tire_f * sigma_fr))));
    F_tot_rl = mu_max * Fz_rl * sin(C_tire * atan(B_tire_r * sigma_rl - E_tire * (B_tire_r * sigma_rl - atan(B_tire_r * sigma_rl))));
    F_tot_rr = mu_max * Fz_rr * sin(C_tire * atan(B_tire_r * sigma_rr - E_tire * (B_tire_r * sigma_rr - atan(B_tire_r * sigma_rr))));
    
    Fx_fl = F_tot_fl * (k_fl / sigma_fl) - C_rr * Fz_fl * tanh(v_hub_fl * 10);
    Fx_fr = F_tot_fr * (k_fr / sigma_fr) - C_rr * Fz_fr * tanh(v_hub_fr * 10);
    Fx_rl = F_tot_rl * (k_rl / sigma_rl) - C_rr * Fz_rl * tanh(v_hub_rl * 10);
    Fx_rr = F_tot_rr * (k_rr / sigma_rr) - C_rr * Fz_rr * tanh(v_hub_rr * 10);
    Fx_vec = [Fx_fl, Fx_fr, Fx_rl, Fx_rr];
    
    Fy_fl = F_tot_fl * (tan(alpha_fl) / sigma_fl);
    Fy_fr = F_tot_fr * (tan(alpha_fr) / sigma_fr);
    Fy_rl = F_tot_rl * (tan(alpha_rl) / sigma_rl);
    Fy_rr = F_tot_rr * (tan(alpha_rr) / sigma_rr);
    Fy_vec = [Fy_fl, Fy_fr, Fy_rl, Fy_rr];
    
    % ---------------------------------------------------------------------
    % 5. CHASSIS & WHEEL INTEGRATORS
    % ---------------------------------------------------------------------
    w_fl_dot = (-abs(Tf_f / 2) * sign(w_fl) - Fx_fl * Rw) / Iw;
    w_fr_dot = (-abs(Tf_f / 2) * sign(w_fr) - Fx_fr * Rw) / Iw;
    w_rl_dot = (Trl_m * G - abs(Trl_f) * sign(w_rl) - Fx_rl * Rw) / Iw;
    w_rr_dot = (Trr_m * G - abs(Trr_f) * sign(w_rr) - Fx_rr * Rw) / Iw;
    w_dot_vec = [w_fl_dot, w_fr_dot, w_rl_dot, w_rr_dot];
    w_vec = [w_fl, w_fr, w_rl, w_rr];
    
    sum_Fx = (Fx_fl + Fx_fr) * cos(delta) - (Fy_fl + Fy_fr) * sin(delta) + Fx_rl + Fx_rr;
    vx_dot = (sum_Fx - F_aero_drag) / m + vy * r;
    
    sum_Fy = (Fy_fl + Fy_fr) * cos(delta) + (Fx_fl + Fx_fr) * sin(delta) + Fy_rl + Fy_rr;
    vy_dot = sum_Fy / m - vx_safe * r;
    
    M_front = lf * ((Fy_fl + Fy_fr) * cos(delta) + (Fx_fl + Fx_fr) * sin(delta));
    M_rear  = -lr * (Fy_rl + Fy_rr);
    M_tv    = (Fx_rr - Fx_rl) * (tw / 2); 
    r_dot  = (M_front + M_rear + M_tv) / Iz;
    
    X_dot   = vx_safe * cos(psi) - vy * sin(psi);
    Y_dot   = vx_safe * sin(psi) + vy * cos(psi);
    psi_dot = r;
    s_dot   = vx_safe;
    
    % ---------------------------------------------------------------------
    % 6. THERMALS & SOC (R-INT BATTERY MODEL)
    % ---------------------------------------------------------------------
    P_mech = (Trr_m + Trl_m) * G * (vx_safe / Rw);
    P_elec = P_mech; 
    
    if P_mech > 500
        P_elec = P_mech / 0.90; 
    elseif P_mech < -500
        P_elec = P_mech * 0.90; 
    end
    
    V_oc = veh_params.V_pack; 
    R_int = 0.015;            
    
    discriminant = V_oc^2 - 4 * R_int * P_elec;
    
    if discriminant < 0
        discriminant = 0;
    end
    
    I_curr = (V_oc - sqrt(discriminant)) / (2 * R_int);
    
    % NEW OUTPUTS
    I_batt = I_curr;
    Pwr_Elec = P_elec;
    
    SOC_dot = -I_curr / (veh_params.Cap_Ah * 3600);
    
    T_batt_dot = ((I_curr^2) * R_int - veh_params.hA_cool_batt * (T_batt - veh_params.T_coolant_batt)) / (veh_params.m_batt * veh_params.cp_batt);
    T_mot_dot  = (abs(P_elec - P_mech) - veh_params.hA_cool_motor * (T_motor - veh_params.T_ambient)) / (veh_params.m_motor * veh_params.cp_motor);
end
